simulink model "analit"  (Simulink 7.4)
settings: Solver=ode45  StartTime=0.0  StopTime=5.0  RelTol=1e-3
settings Model: Creator=bukova.2018  LastModifiedBy=bukova.2018

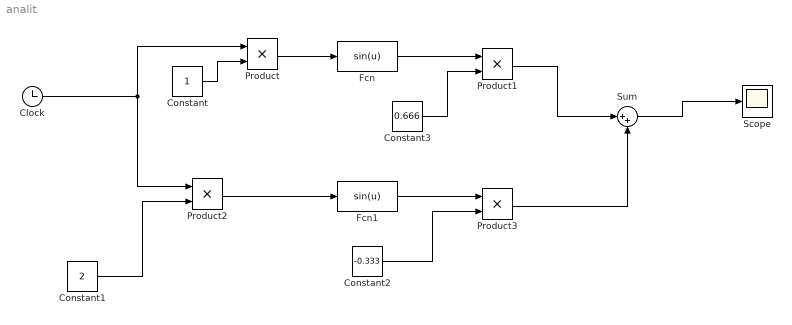
== system analit ==
  Clock : Clock
      settings: Decimation=10
  Constant : Constant  OutDataType=fixdt(1, 16)  OutScaling=2^0
  Constant1 : Constant  Value=2  OutDataType=fixdt(1, 16)  OutScaling=2^0
  Constant2 : Constant  Value=-0.333  OutDataType=fixdt(1, 16)  OutScaling=2^0
  Constant3 : Constant  Value=0.666  OutDataType=fixdt(1, 16)  OutScaling=2^0
  Fcn : Fcn  Expr=sin(u)
  Fcn1 : Fcn  Expr=sin(u)
  Product{,1..3} (4 alike) : Product  OutDataType=fixdt(1, 16)  OutScaling=2^0  RndMeth=Zero
  Scope : Scope
      settings: TimeRange=0.001770760367969082  YMin=-1.610852344418818  YMax=-1.604417623960272
  Sum : Sum  Inputs=|++  OutDataType=fixdt(1, 16)  OutScaling=2^0
  wires:
  Clock/1 -> Product/1, Product2/1
  Constant1/1 -> Product2/2
  Constant/1 -> Product/2
  Product/1 -> Fcn/1
  Fcn/1 -> Product1/1
  Product1/1 -> Sum/1
  Product3/1 -> Sum/2
  Constant3/1 -> Product1/2
  Constant2/1 -> Product3/2
  Fcn1/1 -> Product3/1
  Product2/1 -> Fcn1/1
  Sum/1 -> Scope/1
